simulink model "Problem3"  (R2020a)
settings: Solver=VariableStepAuto  StartTime=0.0  StopTime=10.0  RelTol=1e-3
settings Model: Creator=tanu  LastModifiedBy=tanu

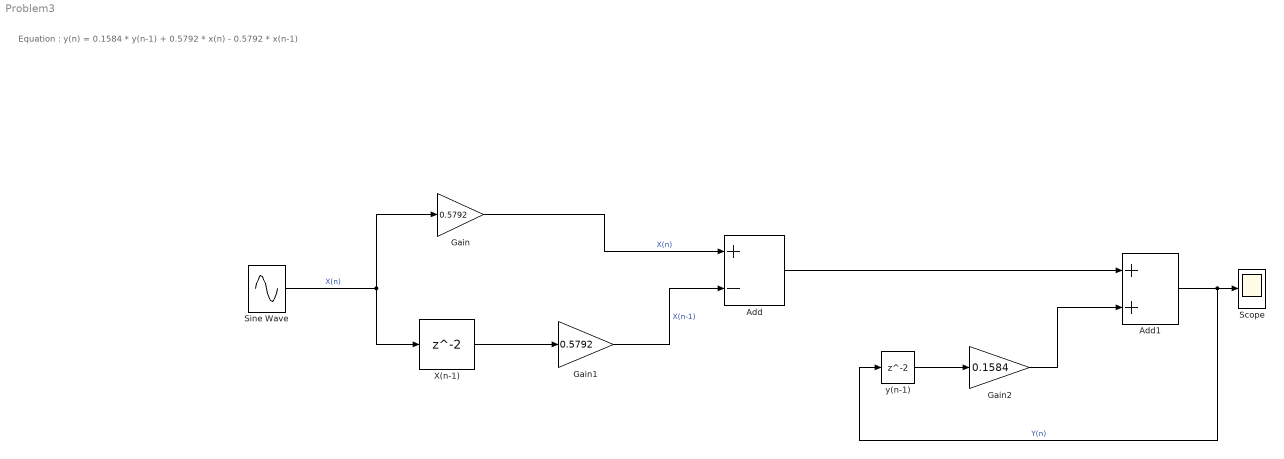
== system Problem3 ==
  note: Equation :
      | y(n) = 0.1584 * y(n-1) + 0.5792 * x(n) - 0.5792 * x(n-1)
  Add : Sum  Inputs=+-
  Add1 : Sum
  Gain : Gain  Gain=0.5792
  Gain1 : Gain  Gain=0.5792
  Gain2 : Gain  Gain=0.1584
  Scope : Scope
  Sine Wave : Sin  SampleTime=0
  X(n-1) : Delay
  y(n-1) : Delay
  wires:
  Gain/1 -> Add/1  "X(n)"
  X(n-1)/1 -> Gain1/1
  Gain1/1 -> Add/2  "X(n-1)"
  Add/1 -> Add1/1
  y(n-1)/1 -> Gain2/1
  Gain2/1 -> Add1/2
  Add1/1 -> y(n-1)/1, Scope/1  "Y(n)"
  Sine Wave/1 -> X(n-1)/1, Gain/1  "X(n)"
